simulink model "InverseDynamics"  (R2024b)
settings: Solver=VariableStepAuto  StartTime=0.0  StopTime=10.0  RelTol=1e-3
undefined symbols (not defined in the file or in its folder): b12, b23, g, I2S2, I3S3, L2, LS2, LS3, m2, m3
settings Model: Creator=jakub  LastModifiedBy=jakub

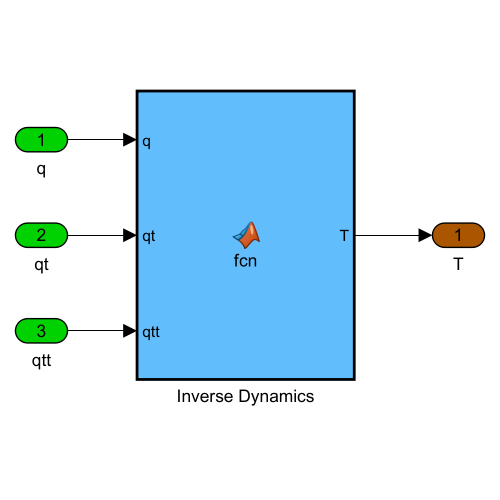
[thumbnail: Simulink's stored preview of the top-level diagram]
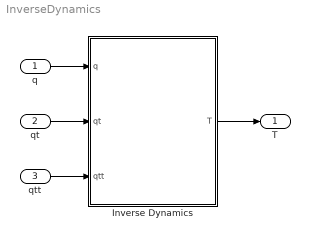
== system InverseDynamics ==
  q : Inport  OutDataTypeStr=double  Unit=rad  PortDimensions=2  SampleTime=0
  qt : Inport  Port=2  OutDataTypeStr=double  Unit=rad/sec  PortDimensions=2  SampleTime=0
  qtt : Inport  Port=3  OutDataTypeStr=double  Unit=rad/sec^2  PortDimensions=2  SampleTime=0
  Inverse Dynamics : MATLAB Function  TreatAsAtomicUnit=on
  T : Outport  OutDataTypeStr=double  Unit=N*m  PortDimensions=2  SampleTime=0
  wires:
  Inverse Dynamics/1(T) -> T/1
  q/1 -> Inverse Dynamics/1(q)
  qt/1 -> Inverse Dynamics/2(qt)
  qtt/1 -> Inverse Dynamics/3(qtt)

== matlab function InverseDynamics/Inverse Dynamics ==
  data: q input double size=[2 1]; T output double size=[2 1]; qt input double size=[2 1]; qtt input double size=[2 1]; m2 parameter double size=1; m3 parameter double size=1; L2 parameter double size=1; LS2 parameter double size=1; LS3 parameter double size=1; g parameter double size=1; I2S2 parameter double size=1; I3S3 parameter double size=1; b12 parameter double size=1; b23 parameter double size=1
function T = fcn(q, qt, qtt, m2, m3, L2, LS2, LS3, g, I2S2, I3S3, b12, b23)
    G2 = m2*g; G3 = m3*g;

% position, velocity
    fi12 = q(1); fi13 = q(2);
    fi12t = qt(1); fi13t = qt(2);



% Mass Matrix
M = [m2*LS2^2 + I2S2 + m3*L2^2, m3*L2*LS3*cos(fi12 - fi13);
     m3*L2*LS3*cos(fi12 - fi13), m3*LS3^2 + I3S3];

% Corriolis and other acc
H = [fi13t^2*m3*L2*LS3*sin(fi12-fi13);
     -fi12t^2*m3*L2*LS3*sin(fi12-fi13)];

% Gravity forces
Q_g = [-G2*LS2*cos(fi12) - G3*L2*cos(fi12); - G3*LS3*cos(fi13)];

% Damping
Q_b = [-b12*fi12t + b23*(fi13t-fi12t);
       -b23*(fi13t-fi12t)];

Q = Q_g + Q_b;

T = M*qtt + H - Q;
